simulink model "SENSIM"  (R2021b)
settings: Solver=FixedStepAuto  StartTime=0.0  StopTime=100.0  FixedStep=0.001  RelTol=1e-3
model workspace (MAT data in the model file):
  Sig = Simulink.Signal
  Sig.DataType = 'auto'
  Sig.Dimensions = -1
  Sig.DimensionsMode = 'auto'
  Sig.Complexity = 'auto'
  Sig.SampleTime = -1
  Sig.SamplingMode = 'auto'
libraries: simulink x2
settings Model: Creator=peter  LastModifiedBy=peter

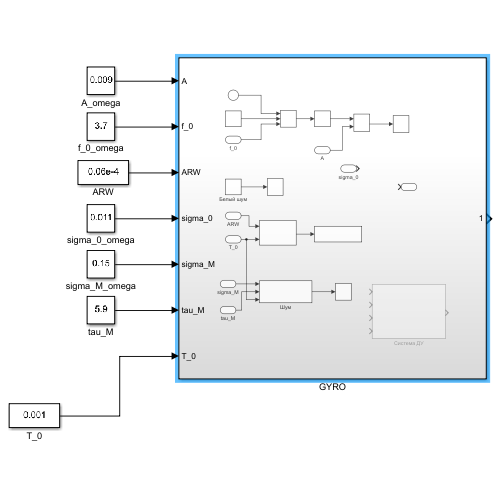
[thumbnail: Simulink's stored preview of the top-level diagram]
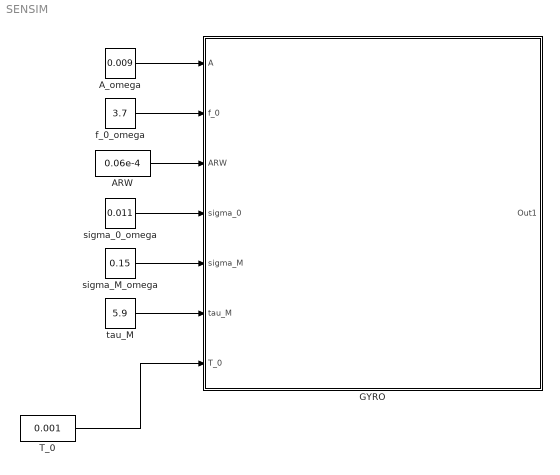
== system SENSIM ==
  ARW : Constant  Value=0.06e-4
  A_omega : Constant  Value=0.009
  GYRO : Subsystem
  T_0 : Constant  Value=0.001
  f_0_omega : Constant  Value=3.7
  sigma_0_omega : Constant  Value=0.011
  sigma_M_omega : Constant  Value=0.15
  tau_M : Constant  Value=5.9
  wires:
  ARW/1 -> GYRO/3(ARW)
  f_0_omega/1 -> GYRO/2(f_0)
  A_omega/1 -> GYRO/1(A)
  sigma_0_omega/1 -> GYRO/4(sigma_0)
  sigma_M_omega/1 -> GYRO/5(sigma_M)
  tau_M/1 -> GYRO/6(tau_M)
  T_0/1 -> GYRO/7(T_0)

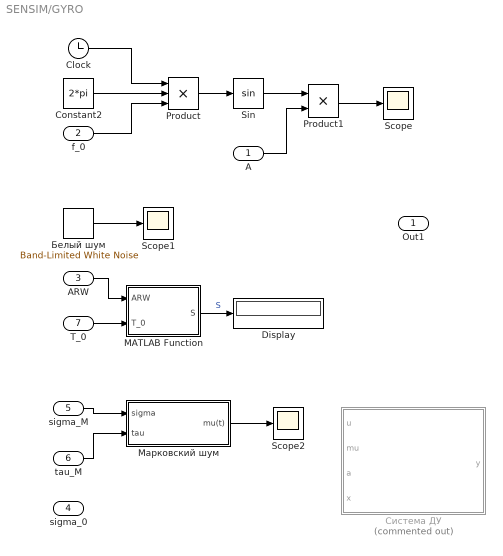
== system SENSIM/GYRO ==
  A : Inport
  f_0 : Inport  Port=2
  ARW : Inport  Port=3
  sigma_0 : Inport  Port=4
  sigma_M : Inport  Port=5
  tau_M : Inport  Port=6
  T_0 : Inport  Port=7
  Clock : Clock
  Constant2 : Constant  Value=2*pi
  Display : Display
  MATLAB Function : MATLAB Function  TreatAsAtomicUnit=on
  Product : Product  Inputs=3
  Product1 : Product
  Scope : Scope
  Scope1 : Scope
  Scope2 : Scope
  Sin : Trigonometry
  Белый шум : simulink/Sources/Band-Limited White Noise  Cov=S  Ts=0.1  seed=[23341]
  Марковский шум : Subsystem
  Система ДУ : MATLAB Function  Commented=on  TreatAsAtomicUnit=on
  Out1 : Outport
  wires:
  Белый шум/1 -> Scope1/1
  MATLAB Function/1(S) -> Display/1  "S"
  Product/1 -> Sin/1
  Constant2/1 -> Product/2
  A/1 -> Product1/2
  ARW/1 -> MATLAB Function/1(ARW)
  Clock/1 -> Product/1
  Sin/1 -> Product1/1
  Product1/1 -> Scope/1
  f_0/1 -> Product/3
  T_0/1 -> MATLAB Function/2(T_0)
  sigma_M/1 -> Марковский шум/1(sigma)
  tau_M/1 -> Марковский шум/2(tau)
  Марковский шум/1(mu(t)) -> Scope2/1

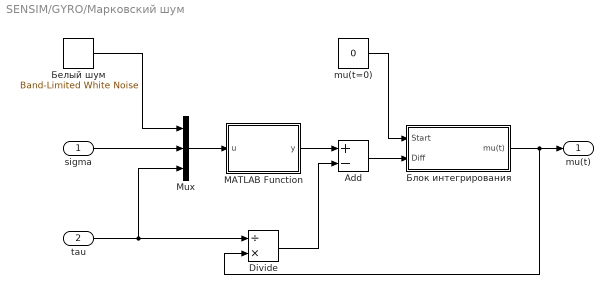
== system SENSIM/GYRO/Марковский шум ==
  sigma : Inport
  tau : Inport  Port=2
  Add : Sum  Inputs=+-
  Divide : Product  Inputs=/*
  MATLAB Function : MATLAB Function  TreatAsAtomicUnit=on
  Mux : Mux  Inputs=3
  mu(t=0) : Constant  Value=0
  Белый шум : simulink/Sources/Band-Limited White Noise  Cov=T_0  Ts=0.1  seed=[23341]
  Блок интегрирования : Subsystem
  mu(t) : Outport
  wires:
  mu(t=0)/1 -> Блок интегрирования/1(Start)
  Блок интегрирования/1(mu(t)) -> Divide/2, mu(t)/1
  sigma/1 -> Mux/2
  tau/1 -> Mux/3, Divide/1
  Add/1 -> Блок интегрирования/2(Diff)
  Divide/1 -> Add/2
  MATLAB Function/1(y) -> Add/1
  Mux/1 -> MATLAB Function/1(u)
  Белый шум/1 -> Mux/1

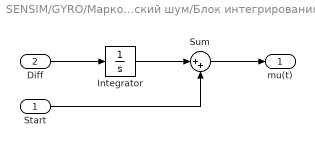
== system SENSIM/GYRO/Марковский шум/Блок интегрирования ==
  Start : Inport
  Diff : Inport  Port=2
  Integrator : Integrator
  Sum : Sum  Inputs=|++
  mu(t) : Outport
  wires:
  Integrator/1 -> Sum/1
  Sum/1 -> mu(t)/1
  Diff/1 -> Integrator/1
  Start/1 -> Sum/2

== matlab function SENSIM/GYRO/Система ДУ ==
  data: u input; y output; mu input; a input; x input
function y = fcn(u,mu,a,x)
    dx_1=x(2);
    dx_2=x(3);
    dx_3=u+mu-a(1)*x(1)-a(2)*x(2)-a(3)*x(3);
y = [dx_1, 
    dx_2, 
    dx_3];

== matlab function SENSIM/GYRO/MATLAB Function ==
  data: ARW input; S output; T_0 input
function S = fcn(ARW,T_0)
    sigma=ARW/sqrt(T_0);
S = sigma^2*T_0;

== matlab function SENSIM/GYRO/Марковский шум/MATLAB Function ==
  data: u input; y output
function y = fcn(u)
    xi=u(1);
    sigma=u(2);
    tau=u(3);
    alpha=1/tau;
    k_f=sigma*sqrt(2*alpha);
y = k_f*xi;
